simulink model "DIsansTOT"  (R2017a)
settings: Solver=VariableStepAuto  StartTime=0.0  StopTime=30  RelTol=1e-3
settings Model: Creator=pc  LastModifiedBy=pc

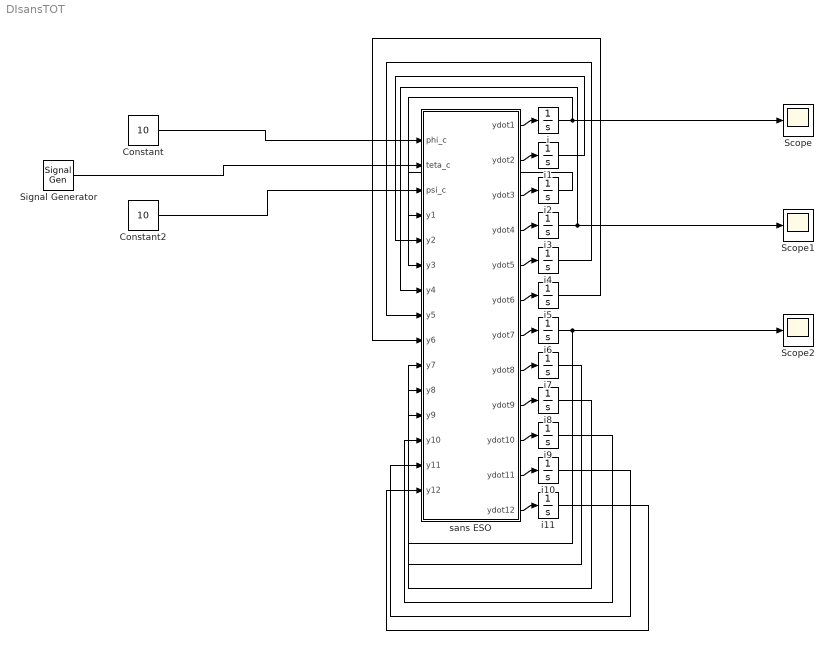
== system DIsansTOT ==
  Constant : Constant  Value=10
  Constant2 : Constant  Value=10
  Scope : Scope
  Scope1 : Scope
  Scope2 : Scope
  Signal Generator : SignalGenerator  WaveForm=square  Amplitude=10  Frequency=0.1
  i{,1..11} (12 alike) : Integrator
  sans ESO : MATLAB Function  TreatAsAtomicUnit=on
  wires:
  sans ESO/1(ydot1) -> i/1
  sans ESO/2(ydot2) -> i1/1
  sans ESO/3(ydot3) -> i2/1
  sans ESO/4(ydot4) -> i3/1
  sans ESO/5(ydot5) -> i4/1
  sans ESO/6(ydot6) -> i5/1
  sans ESO/7(ydot7) -> i6/1
  sans ESO/8(ydot8) -> i7/1
  sans ESO/9(ydot9) -> i8/1
  sans ESO/10(ydot10) -> i9/1
  sans ESO/11(ydot11) -> i10/1
  sans ESO/12(ydot12) -> i11/1
  i/1 -> Scope/1, sans ESO/4(y1)
  i1/1 -> sans ESO/5(y2)
  i2/1 -> sans ESO/6(y3)
  i3/1 -> Scope1/1, sans ESO/7(y4)
  i5/1 -> sans ESO/9(y6)
  i6/1 -> Scope2/1, sans ESO/10(y7)
  i7/1 -> sans ESO/11(y8)
  i8/1 -> sans ESO/12(y9)
  i9/1 -> sans ESO/13(y10)
  i10/1 -> sans ESO/14(y11)
  i11/1 -> sans ESO/15(y12)
  i4/1 -> sans ESO/8(y5)
  Constant/1 -> sans ESO/1(phi_c)
  Signal Generator/1 -> sans ESO/2(teta_c)
  Constant2/1 -> sans ESO/3(psi_c)

== matlab function DIsansTOT/sans ESO ==
  data: phi_c input; teta_c input; psi_c input; y1 input; ydot1 output; y2 input; y3 input; y4 input; y5 input; y6 input; y7 input; y8 input; y9 input; y10 input; y11 input; y12 input; ydot2 output; ydot3 output; ydot4 output; ydot5 output; ydot6 output; ydot7 output; ydot8 output; ydot9 output; ydot10 output; ydot11 output; ydot12 output
function [ydot1,ydot2,ydot3,ydot4,ydot5,ydot6,ydot7,ydot8,ydot9,ydot10,ydot11,ydot12] = fcn(phi_c,teta_c,psi_c,y1,y2,y3,y4,y5,y6,y7,y8,y9,y10,y11,y12)
kd1=6.4;kd2=6.4;kd3=6.4;
kp1=16;kp2=16;kp3=16;
%--------------------------------------------------------------------------
% Ix=12874.8;
% Iy=75673.6;
% Iz=85552.1;
% Ixz=1331.4;
Ix=22682;
Iy=77095;
Iz=95561;
Ixz=1125;
SOM=Ix*Iz-Ixz^2;
c1=((Iy-Iz)*Iz-Ixz^2)/SOM;
c2=((Ix-Iy+Iz)*Ixz)/SOM;
c3=Iz/SOM;
c4=Ixz/SOM;
c5=(Iz-Ix)/Iy;
c6=Ixz/Iy;
c7=1/Iy;
c8=(Ix*(Ix-Iy)+Ixz^2)/SOM;
c9=Ix/SOM;
%--------------------------------------------------------------------------
phi=y1;
teta=y4;
p=y10;
r=y11;
q=y12;
%--------------------------------------------------------------------------
B=[c3+c4*cosd(phi)*tand(teta),c7*sind(phi)*tand(teta),c4+c9*cosd(phi)*tand(teta);
    -c4*sind(phi),c7*cosd(phi),-c9*sind(phi);
    c4*cosd(phi)*(1/cosd(teta)),c7*sind(phi)*(1/cosd(teta)),c9*cosd(phi)*(1/cosd(teta))];
phidot=p+tand(teta)*(q*sind(phi)+r*cosd(phi));
tetadot=q*cosd(phi)-r*sind(phi);
A1=((c1*r+c2*p)*q)+(tetadot/cosd(teta)^2)*(q*sind(phi)+r*cosd(phi))+tand(teta)*((c5*p*r-c6*(p^2-r^2))*sind(phi)+q*(phidot*cosd(phi))+((c8*p-c2*r)*q)*cosd(phi)-r*phidot*sind(phi));
A2=(c5*p*r-c6*(p^2-r^2))*cosd(phi)-phidot*sind(phi)*q-(((c8*p-c2*r)*q)*sind(phi)+phidot*cosd(phi)*r);
A3=((c5*p*r-c6*(p^2-r^2))*sind(phi)+phidot*cosd(phi)*q+((c8*p-c2*r)*q)*cosd(phi)-phidot*sind(phi)*r)*cosd(teta)/cosd(teta)^2+(tetadot*sind(teta)*(q*sind(phi)+r*cosd(phi)))/cosd(teta)^2;
A=[A1;A2;A3];
%--------------------------------------------------------------------------
Bdot=[c4*cosd(phi)*(tand(teta)^2 + 1)*tetadot - c4*sind(phi)*tand(teta)*phidot,c7*cosd(phi)*tand(teta)*phidot + c7*sind(phi)*(tand(teta)^2 + 1)*tetadot,c9*cosd(phi)*(tand(teta)^2 + 1)*tetadot - c9*sind(phi)*tand(teta)*phidot;
     -c4*cosd(phi)*phidot,-c7*sind(phi)*phidot,-c9*cosd(phi)*phidot;
     (c4*cosd(phi)*sind(teta)*tetadot)/cosd(teta)^2 - (c4*sind(phi)*phidot)/cosd(teta), (c7*cosd(phi)*phidot)/cosd(teta) + (c7*sind(phi)*sind(teta)*tetadot)/cosd(teta)^2, (c9*cosd(phi)*sind(teta)*tetadot)/cosd(teta)^2 - (c9*sind(phi)*phidot)/cosd(teta)];
%--------------------------------------------------------------------------
pp=inv(B);
L=pp(1,:)*[(kp1*(phi_c-y1)-kd1*y2)-A1;((kp2*(teta_c-y4)-kd2*y5)-A2);((kp3*(psi_c-y7)-kd3*y8)-A3)];
M=pp(2,:)*[(kp1*(phi_c-y1)-kd1*y2)-A1;((kp2*(teta_c-y4)-kd2*y5)-A2);((kp3*(psi_c-y7)-kd3*y8)-A3)];
N=pp(3,:)*[(kp1*(phi_c-y1)-kd1*y2)-A1;((kp2*(teta_c-y4)-kd2*y5)-A2);((kp3*(psi_c-y7)-kd3*y8)-A3)];
pdot=(c1*r+c2*p)*q+c3*L+c4*N;
rdot=(c8*p-c2*r)*q+c4*L+c9*N;
qdot=c5*p*r-c6*(p^2-r^2)+c7*M;

phidotdot=pdot+(tetadot/cosd(teta)^2)*(q*sind(phi)+r*cosd(phi))+tand(teta)*(qdot*sind(phi)+q*(phidot*cosd(phi))+rdot*cosd(phi)-r*phidot*sind(phi));
tetadotdot=qdot*cosd(phi)-phidot*sind(phi)*q-(rdot*sind(phi)+phidot*cosd(phi)*r);

A1dot=(c1*rdot+c2*pdot)*q+qdot*(c1*r+c2*p)+(tetadotdot*cosd(teta)^2+2*tetadot^2*sind(teta)*cosd(teta))/cosd(teta)^4*(q*sind(phi)+r*cosd(phi))+(qdot*sind(phi)+phidot*cosd(phi)*q+rdot*cosd(phi)-phidot*sind(phi)*r)*(tetadot/cosd(teta)^2)+(tetadot/cosd(teta)^2)*((c5*p*r-c6*(p^2-r^2))*sind(phi)+q*(phidot*cosd(phi))+((c8*p-c2*r)*q)*cosd(phi)-r*phidot*sind(phi))+((c5*p*r-c6*(p^2-r^2))*phidot*cosd(phi)+(c5*(pdot*r+rdot*p)-c6*(2*p*pdot-2*r*rdot))*sind(phi)+(qdot*phidot+phidotdot*q)*cosd(phi)-phidot*sind(phi)*q*phidot+(c8*pdot-c2*rdot)*q*cosd(phi)+(qdot*cosd(phi)-phidot*sind(phi)*q)*(c8*p-c2*r)-((rdot*phidot+phidotdot*r)*sind(phi)+phidot*cosd(phi)*r*phidot))*tand(teta);
A2dot=(c5*(pdot*r+rdot*p)-c6*(2*p*pdot-2*r*rdot))*cosd(phi)-phidot*sind(phi)*(c5*p*r-c6*(p^2-r^2))-((phidotdot*q+qdot*phidot)*sind(phi)+phidot*cosd(phi)*phidot*q)-(((c8*pdot-c2*rdot)*q+qdot*(c8*p-c2*r))*sind(phi)+phidot*cosd(phi)*((c8*p-c2*r)*q)+(phidotdot*r+rdot*phidot)*cosd(phi)-phidot*sind(phi)*phidot*r);
A3dot=((((c5*(pdot*r+rdot*p)-c6*(2*p*pdot-2*r*rdot))*sind(phi)+phidot*cosd(phi)*(c5*p*r-c6*(p^2-r^2))+(phidotdot*cosd(phi)-phidot*sind(phi)*phidot)*q+qdot*phidot*cosd(phi)+((c8*pdot-c2*rdot)*q+qdot*(c8*p-c2*r))*cosd(phi)-phidot*sind(phi)*((c8*p-c2*r)*q)-((phidotdot*sind(phi)+phidot*cosd(phi)*phidot)*r+rdot*phidot*sind(phi)))*cosd(teta)-tetadot*sind(teta)*((c5*p*r-c6*(p^2-r^2))*sind(phi)+phidot*cosd(phi)*q+(c5*p*r-c6*(p^2-r^2))*cosd(phi)-phidot*sind(phi)*r))*cosd(teta)^2+2*tetadot*cosd(teta)*sind(teta)*((c5*p*r-c6*(p^2-r^2))*sind(phi)+phidot*cosd(phi)*q+((c8*p-c2*r)*q)*cosd(phi)-phidot*sind(phi)*r)*cosd(teta))/cosd(teta)^4+(((tetadotdot*sind(teta)+tetadot*cosd(teta)*tetadot)*(q*sind(phi)+r*cosd(phi))+(qdot*sind(phi)+phidot*cosd(phi)*q+rdot*cosd(phi)-phidot*sind(phi)*r)*tetadot*sind(teta))*cosd(teta)^2+2*tetadot*cosd(teta)*sind(teta)*(tetadot*sind(teta)*(q*sind(phi)+r*cosd(phi))))/cosd(teta)^4;
Adot=[A1dot;A2dot;A3dot];
%--------------------------------------------------------------------------
u=[L;M;N];
ppdot=[ 0, -(c4*cosd(phi)*phidot)/(c4^2*cosd(phi)^2 + c4^2*sind(phi)^2 - c3*c9*cosd(phi)^2 - c3*c9*sind(phi)^2), (cosd(teta)*(c9*cosd(phi)^2*(tand(teta)^2 + 1)*tetadot - c4*sind(phi)*phidot + c9*sind(phi)^2*(tand(teta)^2 + 1)*tetadot))/(c4^2*cosd(phi)^2 + c4^2*sind(phi)^2 - c3*c9*cosd(phi)^2 - c3*c9*sind(phi)^2) - (sind(teta)*tetadot*(c9*tand(teta)*cosd(phi)^2 + c4*cosd(phi) + c9*tand(teta)*sind(phi)^2))/(c4^2*cosd(phi)^2 + c4^2*sind(phi)^2 - c3*c9*cosd(phi)^2 - c3*c9*sind(phi)^2);
        0,                                                    -(sind(phi)*phidot)/(c7*cosd(phi)^2 + c7*sind(phi)^2),                                                                                                                                                                                                                                                                                             (cosd(phi)*cosd(teta)*phidot)/(c7*cosd(phi)^2 + c7*sind(phi)^2) - (sind(phi)*sind(teta)*tetadot)/(c7*cosd(phi)^2 + c7*sind(phi)^2);
        0,  (c3*cosd(phi)*phidot)/(c4^2*cosd(phi)^2 + c4^2*sind(phi)^2 - c3*c9*cosd(phi)^2 - c3*c9*sind(phi)^2), (sind(teta)*tetadot*(c4*tand(teta)*cosd(phi)^2 + c3*cosd(phi) + c4*tand(teta)*sind(phi)^2))/(c4^2*cosd(phi)^2 + c4^2*sind(phi)^2 - c3*c9*cosd(phi)^2 - c3*c9*sind(phi)^2) - (cosd(teta)*(c4*cosd(phi)^2*(tand(teta)^2 + 1)*tetadot - c3*sind(phi)*phidot + c4*sind(phi)^2*(tand(teta)^2 + 1)*tetadot))/(c4^2*cosd(phi)^2 + c4^2*sind(phi)^2 - c3*c9*cosd(phi)^2 - c3*c9*sind(phi)^2)];
v=[(kp1*(phi_c-y1)-kd1*y2);(kp2*(teta_c-y4)-kd2*y5);(kp3*(psi_c-y7)-kd3*y8)];
vdot=[-kp1*y2-kd1*(y3+kp1*phi_c);-kp2*y5-kd2*(y6+kp2*teta_c);-kp3*y8-kd3*(y9+kp3*psi_c)];
udot=ppdot*(v-A)+pp*(vdot-Adot);
%--------------------------------------------------------------------------
ydot1=y2;   
%ydot(2)=A1+B(1,:)*[L;M;N];
ydot2=y3+kp1*phi_c;
ydot3=A1dot+Bdot(1,:)*u+B(1,:)*udot;
%--------------------------------------------------------------------------
ydot4=y5;   
%ydot(4)=A2+B(2,:)*[L;M;N];  
ydot5=y6+kp2*teta_c;
ydot6=A2dot+Bdot(2,:)*u+B(2,:)*udot;
%--------------------------------------------------------------------------
ydot7=y8;   
%ydot(6)=A3+B(3,:)*[L;M;N];
ydot8=y9+kp3*psi_c;
ydot9=A3dot+Bdot(3,:)*u+B(3,:)*udot;
%--------------------------------------------------------------------------
ydot10=(c1*r+c2*p)*q+c3*L+c4*N;  %=pdot
ydot11=(c8*p-c2*r)*q+c4*L+c9*N;  %=rdot
ydot12=c5*p*r-c6*(p^2-r^2)+c7*M; %=qdot
end
